simulink model "Assignment_1"  (R2022b)
settings: Solver=FixedStepAuto  StartTime=0.0  StopTime=10.0  FixedStep=1e-3  RelTol=1e-3  EnableMultiTasking=on
undefined symbols (not defined in the file): D0, D1, D10, D11, D12, D13, D2, D3, D5, D6, D8, D9, PTA0, PTA1, PTA2, PTB9, PTC16, PTC17, PTC2, PTC4, PTD0, PTD1, PTD2, PTD3
libraries: frdmk64flib x12
settings Model: ExtModeTrigDuration=5  Creator=aldenluscher  LastModifiedBy=andre
settings OptimizationCC: EnhancedBackFolding=on  PassReuseOutputArgsAs=Individual arguments  ZeroExternalMemoryAtStartup=off  ZeroInternalMemoryAtStartup=off  MaxStackSize=64  OptimizeBlockOrder=speed  DifferentSizesBufferReuse=on  OptimizationCustomize=off  EfficientTunableParamExpr=on
settings DebuggingCC: ParameterTunabilityLossMsg=error
settings HardwareCC: ProdBitPerPointer=32  ProdBitPerSizeT=32  ProdBitPerPtrDiffT=32  ProdLargestAtomicInteger=Long  ProdLargestAtomicFloat=Double  ProdWordSize=32  ProdHWDeviceType=ARM Compatible->ARM Cortex
settings SFSimCC: MATLABDynamicMemAlloc=off
settings RTWCC: Description=Embedded Coder  SystemTargetFile=ert.tlc  HardwareBoard=NXP FRDM-K64F  TLCOptions="-aInlineSetEventsForThisBaseRateFcn=TLC_FALSE -aSuppressMultiTaskScheduler=TLC_FALSE  -aRateBasedStepFcn=0"  TemplateMakefile=ert_default_tmf  Toolchain=GNU Tools for ARM Embedded Processors
settings CodeAppCC: ForceParamTrailComments=on  IgnoreCustomStorageClasses=off  OperatorAnnotations=on  SimulinkDataObjDesc=on  SFDataObjDesc=on  InsertBlockDesc=on
settings ERTTargetCC: ExtModeTransport=4  ExtModeMexFile=sendToCommService

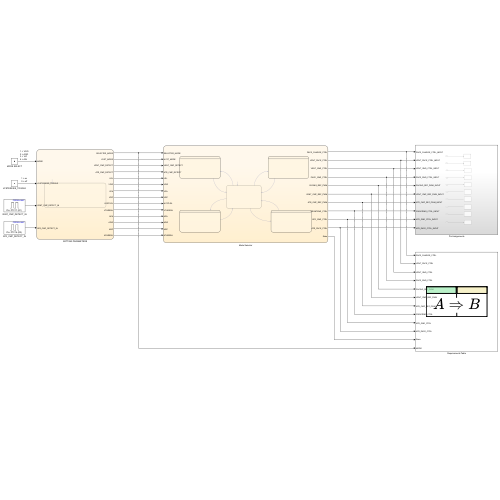
[thumbnail: Simulink's stored preview of the top-level diagram]
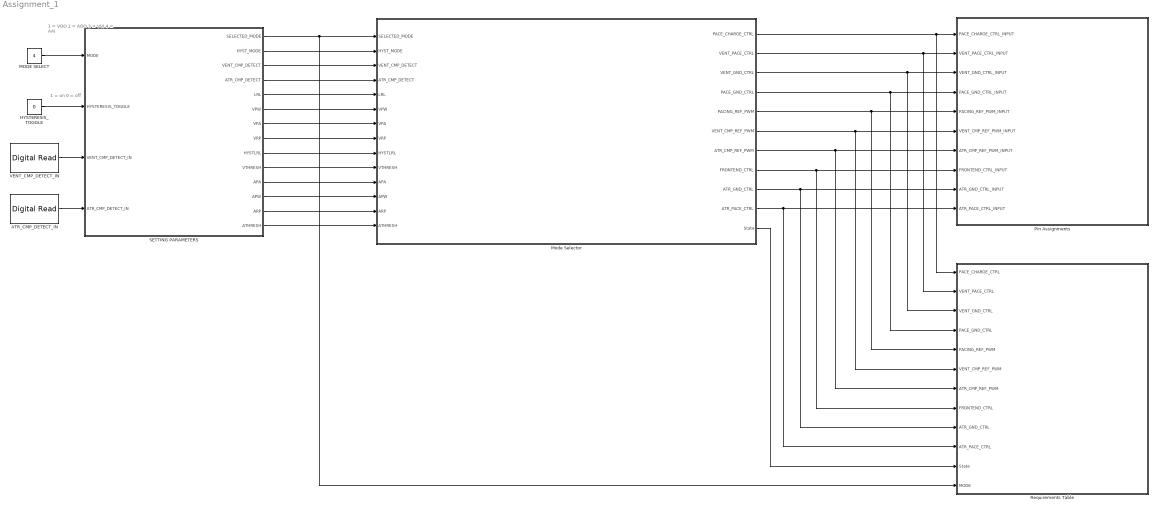
== system Assignment_1 ==
  note: 1 = VOO
      | 2 = AOO
      | 3 = VVI
      | 4 = AAI
  note: 1 = on
      | 0 = off
  ATR_CMP_DETECT_IN : frdmk64flib/Digital Read  Whichpin=PTC16 (D0)  SampleTime=-1
  HYSTERESIS_TOGGLE : Constant  Value=0
  MODE SELECT : Constant  Value=4  OutDataTypeStr=int8
  Mode Selector : Stateflow chart  TreatAsAtomicUnit=on
      settings: PortSchema="{\"entries\":[{\"content\":{\"sides\":[{\"content\":{\"connectorIds\":[\"In7\",\"In9\",\"In6\",\"In14\",\"In8\",\"In3\",\"In4\",\"In2\",\"In5\",\"In1\",\"In10\",\"In11\",\"In12\",\"In13\"]},\"type\":\"ConnectorPlacement.EquallySpacedRectSide\",\"uuid\":\"804be3be-5f9e-4b62-b5c8-dc084235daae\"},{\"content\":{\"connectorIds\":[\"Out1\",\"Out2\",\"Out3\",\"Out4\",\"Out5\",\"Out6\",\"Out11\",\"Out7\",\"Out8\",\"Out9\",\"Out10\"],\"side\":\"RIGHT\"},\"type\":\"ConnectorPlacement.EquallySpacedRectSide\",\"uuid\":\"906acfdb-1dc8-44fd-8d51-f28f98719a27\"},{\"content\":{\"connectorIds\":[],\"side\":\"TOP\"},\"type\":\"ConnectorPlacement.EquallySpacedRectSide\",\"uuid\":\"8d057b55-2cbd-487f-8484-177f9fa59c90\"}]},\"type\":\"ConnectorPlacement.EquallySpacedConnector\",\"uuid\":\"d5bd6f86-9a36-412f-a1f0-e96663509123\"}],\"packageUris\":[\"http://schema.mathworks.com/mf0/Connector/R2020b\"],\"version\":\"1.0\"}"
  Pin Assignments : Subsystem
  Requirements Table : Requirements Table  TreatAsAtomicUnit=on
  SETTING PARAMETERS : Stateflow chart  TreatAsAtomicUnit=on
      settings: PortSchema="{\"entries\":[{\"content\":{\"sides\":[{\"content\":{\"connectorIds\":[\"In1\",\"In2\",\"In3\",\"In4\"]},\"type\":\"ConnectorPlacement.EquallySpacedRectSide\",\"uuid\":\"3aca0bd7-629a-4c5c-b565-6ed0578fed9d\"},{\"content\":{\"connectorIds\":[\"Out7\",\"Out9\",\"Out6\",\"Out14\",\"Out8\",\"Out3\",\"Out4\",\"Out2\",\"Out5\",\"Out1\",\"Out10\",\"Out11\",\"Out12\",\"Out13\"],\"side\":\"RIGHT\"},\"type\":\"ConnectorPlacement.EquallySpacedRectSide\",\"uuid\":\"ab26bc13-3a59-4dfe-8b46-0847370ad477\"},{\"content\":{\"connectorIds\":[],\"side\":\"TOP\"},\"type\":\"ConnectorPlacement.EquallySpacedRectSide\",\"uuid\":\"fc5ed4b5-9a01-4cf9-a838-586958f03313\"}]},\"type\":\"ConnectorPlacement.EquallySpacedConnector\",\"uuid\":\"c620314d-9c7d-46a3-b2b8-c6bca5c5944e\"}],\"packageUris\":[\"http://schema.mathworks.com/mf0/Connector/R2020b\"],\"version\":\"1.0\"}"
  VENT_CMP_DETECT_IN : frdmk64flib/Digital Read  Whichpin=PTC17 (D1)  SampleTime=-1
  wires:
  MODE SELECT/1 -> SETTING PARAMETERS/1(MODE)
  HYSTERESIS_TOGGLE/1 -> SETTING PARAMETERS/2(HYSTERESIS_TOGGLE)
  VENT_CMP_DETECT_IN/1 -> SETTING PARAMETERS/3(VENT_CMP_DETECT_IN)
  Mode Selector/4(PACE_GND_CTRL) -> Requirements Table/4(PACE_GND_CTRL), Pin Assignments/4(PACE_GND_CTRL_INPUT)
  Mode Selector/7(FRONTEND_CTRL) -> Pin Assignments/8(FRONTEND_CTRL_INPUT), Requirements Table/8(FRONTEND_CTRL)
  Mode Selector/5(PACING_REF_PWM) -> Requirements Table/5(PACING_REF_PWM), Pin Assignments/5(PACING_REF_PWM_INPUT)
  Mode Selector/1(PACE_CHARGE_CTRL) -> Requirements Table/1(PACE_CHARGE_CTRL), Pin Assignments/1(PACE_CHARGE_CTRL_INPUT)
  Mode Selector/3(VENT_GND_CTRL) -> Requirements Table/3(VENT_GND_CTRL), Pin Assignments/3(VENT_GND_CTRL_INPUT)
  Mode Selector/6(VENT_CMP_REF_PWM) -> Requirements Table/6(VENT_CMP_REF_PWM), Pin Assignments/6(VENT_CMP_REF_PWM_INPUT)
  Mode Selector/2(VENT_PACE_CTRL) -> Requirements Table/2(VENT_PACE_CTRL), Pin Assignments/2(VENT_PACE_CTRL_INPUT)
  SETTING PARAMETERS/1(VTHRESH) -> Mode Selector/1(VTHRESH)
  SETTING PARAMETERS/2(VRP) -> Mode Selector/2(VRP)
  SETTING PARAMETERS/3(VPW) -> Mode Selector/3(VPW)
  SETTING PARAMETERS/4(VPA) -> Mode Selector/4(VPA)
  SETTING PARAMETERS/5(HYSTLRL) -> Mode Selector/5(HYSTLRL)
  SETTING PARAMETERS/6(VENT_CMP_DETECT) -> Mode Selector/6(VENT_CMP_DETECT)
  SETTING PARAMETERS/7(SELECTED_MODE) -> Requirements Table/12(MODE), Mode Selector/7(SELECTED_MODE)
  SETTING PARAMETERS/8(LRL) -> Mode Selector/8(LRL)
  SETTING PARAMETERS/9(HYST_MODE) -> Mode Selector/9(HYST_MODE)
  SETTING PARAMETERS/10(APA) -> Mode Selector/10(APA)
  SETTING PARAMETERS/11(APW) -> Mode Selector/11(APW)
  Mode Selector/8(ATR_GND_CTRL) -> Pin Assignments/9(ATR_GND_CTRL_INPUT), Requirements Table/9(ATR_GND_CTRL)
  Mode Selector/9(ATR_PACE_CTRL) -> Pin Assignments/10(ATR_PACE_CTRL_INPUT), Requirements Table/10(ATR_PACE_CTRL)
  Mode Selector/10(State) -> Requirements Table/11(State)
  ATR_CMP_DETECT_IN/1 -> SETTING PARAMETERS/4(ATR_CMP_DETECT_IN)
  SETTING PARAMETERS/12(ARP) -> Mode Selector/12(ARP)
  SETTING PARAMETERS/13(ATHRESH) -> Mode Selector/13(ATHRESH)
  SETTING PARAMETERS/14(ATR_CMP_DETECT) -> Mode Selector/14(ATR_CMP_DETECT)
  Mode Selector/11(ATR_CMP_REF_PWM) -> Requirements Table/7(ATR_CMP_REF_PWM), Pin Assignments/7(ATR_CMP_REF_PWM_INPUT)

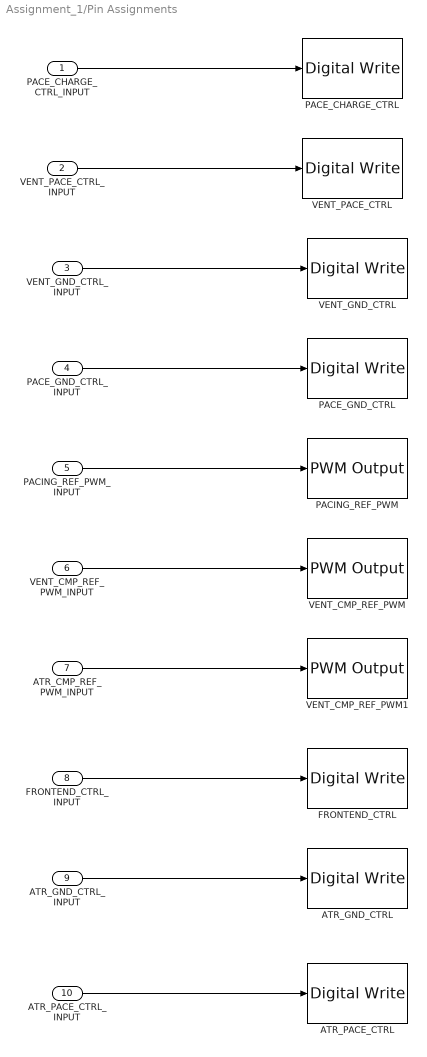
== system Assignment_1/Pin Assignments ==
  PACE_CHARGE_CTRL_INPUT : Inport
  VENT_PACE_CTRL_INPUT : Inport  Port=2
  VENT_GND_CTRL_INPUT : Inport  Port=3
  PACE_GND_CTRL_INPUT : Inport  Port=4
  PACING_REF_PWM_INPUT : Inport  Port=5
  VENT_CMP_REF_PWM_INPUT : Inport  Port=6
  ATR_CMP_REF_PWM_INPUT : Inport  Port=7
  FRONTEND_CTRL_INPUT : Inport  Port=8
  ATR_GND_CTRL_INPUT : Inport  Port=9
  ATR_PACE_CTRL_INPUT : Inport  Port=10
  ATR_GND_CTRL : frdmk64flib/Digital Write  Whichpin=PTD2 (D11)
  ATR_PACE_CTRL : frdmk64flib/Digital Write  Whichpin=PTA0 (D8)
  FRONTEND_CTRL : frdmk64flib/Digital Write  Whichpin=PTD1 (D13)
  PACE_CHARGE_CTRL : frdmk64flib/Digital Write  Whichpin=PTB9 (D2)
  PACE_GND_CTRL : frdmk64flib/Digital Write  Whichpin=PTD0 (D10)
  PACING_REF_PWM : frdmk64flib/PWM Output  Whichpin=PTA2 (D5)  InitialFrequency=2000  InitialDutyCycle=0
  VENT_CMP_REF_PWM : frdmk64flib/PWM Output  Whichpin=PTA1 (D3)  InitialFrequency=2000  InitialDutyCycle=0
  VENT_CMP_REF_PWM1 : frdmk64flib/PWM Output  Whichpin=PTC2 (D6)  InitialFrequency=2000  InitialDutyCycle=0
  VENT_GND_CTRL : frdmk64flib/Digital Write  Whichpin=PTD3 (D12)
  VENT_PACE_CTRL : frdmk64flib/Digital Write  Whichpin=PTC4 (D9)
  wires:
  VENT_PACE_CTRL_INPUT/1 -> VENT_PACE_CTRL/1
  PACE_GND_CTRL_INPUT/1 -> PACE_GND_CTRL/1
  PACE_CHARGE_CTRL_INPUT/1 -> PACE_CHARGE_CTRL/1
  PACING_REF_PWM_INPUT/1 -> PACING_REF_PWM/1
  VENT_GND_CTRL_INPUT/1 -> VENT_GND_CTRL/1
  VENT_CMP_REF_PWM_INPUT/1 -> VENT_CMP_REF_PWM/1
  FRONTEND_CTRL_INPUT/1 -> FRONTEND_CTRL/1
  ATR_GND_CTRL_INPUT/1 -> ATR_GND_CTRL/1
  ATR_PACE_CTRL_INPUT/1 -> ATR_PACE_CTRL/1
  ATR_CMP_REF_PWM_INPUT/1 -> VENT_CMP_REF_PWM1/1

== stateflow chart Assignment_1/SETTING PARAMETERS ==
  state Parameters_
    SELECTED_MODE = MODE; % Pacing Mode
    HYST_MODE = HYSTERESIS_TOGGLE; % Toggles On/Off Hysteresis (1 = on, 0 = off)
    VENT_CMP_DETECT = VENT_CMP_DETECT_IN; % Input value read from D1 pin
    ATR_CMP_DETECT = ATR_CMP_DETECT_IN;% Input value read from D0 pin
    LRL = 120; %  Lower Rate Limit (e.g. 120ppm)
    HYSTLRL = 50; % Ventricle Hysteresis Lower Rate Limit (e.g. 50ppm)
    VPW = 1; % Ventricle Pulse Width
    VPA = 3.5; % Ventricle Pulse Amplitude (as voltage from 1-5V)
    VRP = 300; % Ventricle Refractory Period (msec)
    VTHRESH = 70; % Ventricle Pulse Detection Threshold as PWM Value (e.g 70% of 5V)
    APW = 1; % Atrial Pulse Width
    APA = 3.5; % Atrial Pulse Amplitude (as voltage from 1-5V)
    ARP = 300; % Atrial Refractory Period (msec)
    ATHRESH = 70; % Atrial Pulse Detection Threshold as a PWM Value (e.g. 70% of 5V)
  (default) -> Parameters_
  data: PACING_PERIOD local; MODE input int8 [1..4]; HYSTERESIS_TOGGLE input; VENT_CMP_DETECT_IN input; VTHRESH output; VRP output; VPW output; VPA output; HYSTLRL output; VENT_CMP_DETECT output; SELECTED_MODE output; LRL output; HYST_MODE output; APA output; APW output; ATR_CMP_DETECT_IN input; ARP output; ATHRESH output; ATR_CMP_DETECT output

== stateflow chart Assignment_1/Requirements Table ==
  (default) -> (junction 1073752893)
  (junction 1073752893) -> (junction 1073752894) : {
      | % SF_REQ_REV_07
      | }
  (junction 1073752894) -> (junction 1073752896) : {
      | % HEADER_ASSIGNMENTS
      |
      | }
  (junction 1073752896) -> (junction 1073752898) : {
      | % START_A_4
      | }
  (junction 1073752898) -> (junction 1073752900) : {
      | }
  (junction 1073752900) -> (junction 1073752902) : {
      | reqtable_assumption((0<= State && State <= 2), 4);
      | }
  (junction 1073752902) -> (junction 1073752904) : {
      | }
  (junction 1073752904) -> (junction 1073752906) : {
      | % END_A_4
      | }
  (junction 1073752906) -> (junction 1073753176) : {
      | % START_A_76
      | }
  (junction 1073753176) -> (junction 1073753178) : {
      | }
  (junction 1073753178) -> (junction 1073753180) : {
      | reqtable_assumption((1<= MODE && MODE <= 4), 76);
      | }
  (junction 1073753180) -> (junction 1073753182) : {
      | }
  (junction 1073753182) -> (junction 1073753184) : {
      | % END_A_76
      | }
  (junction 1073753184) -> (junction 1073752908) : {
      | % START_R_40
      | }
  (junction 1073752908) -> (junction 1073752910) : {
      | }
  (junction 1073752910) -> (junction 1073752912)
  (junction 1073752912) -> (junction 1073752914) [order 1] : [(((MODE) == (1)))]
  (junction 1073752912) -> (junction 1073752956) [order 2]
  (junction 1073752914) -> (junction 1073752916) : {
      | reqtable_postcondition((((ATR_PACE_CTRL) == (0))) && (((ATR_GND_CTRL) == (0))) && (((PACING_REF_PWM) >= (0) && (PACING_REF_PWM) <= (100))) && (((VENT_CMP_REF_PWM) >= (0) && (VENT_CMP_REF_PWM) <= (100))) && (((ATR_CMP_REF_PWM) >= (0) && (ATR_CMP_REF_PWM) <= (100))) && (((FRONTEND_CTRL) == (0))), 'R:1');
      |
      |
      | }
  (junction 1073752916) -> (junction 1073752918) : {
      | }
  (junction 1073752918) -> (junction 1073752920) : {
      | % START_R_16
      | }
  (junction 1073752920) -> (junction 1073752922) : {
      | }
  (junction 1073752922) -> (junction 1073752924)
  (junction 1073752924) -> (junction 1073752926) [order 1] : [(((State) == (0)))]
  (junction 1073752924) -> (junction 1073752932) [order 2]
  (junction 1073752926) -> (junction 1073752928) : {
      | reqtable_postcondition((((PACE_CHARGE_CTRL) == (1))) && (((PACE_GND_CTRL) == (1))) && (((VENT_PACE_CTRL) == (0))) && (((VENT_GND_CTRL) == (1))), 'R:1.1');
      |
      |
      | }
  (junction 1073752928) -> (junction 1073752930) : {
      | }
  (junction 1073752930) -> (junction 1073752932)
  (junction 1073752932) -> (junction 1073752934)
  (junction 1073752934) -> (junction 1073752936) : {
      | % END_R_16
      | }
  (junction 1073752936) -> (junction 1073752938) : {
      | % START_R_22
      | }
  (junction 1073752938) -> (junction 1073752940) : {
      | }
  (junction 1073752940) -> (junction 1073752942)
  (junction 1073752942) -> (junction 1073752944) [order 1] : [(((State) == (1)))]
  (junction 1073752942) -> (junction 1073752950) [order 2]
  (junction 1073752944) -> (junction 1073752946) : {
      | reqtable_postcondition((((PACE_CHARGE_CTRL) == (0))) && (((PACE_GND_CTRL) == (1))) && (((VENT_PACE_CTRL) == (1))) && (((VENT_GND_CTRL) == (0))), 'R:1.2');
      |
      |
      | }
  (junction 1073752946) -> (junction 1073752948) : {
      | }
  (junction 1073752948) -> (junction 1073752950)
  (junction 1073752950) -> (junction 1073752952)
  (junction 1073752952) -> (junction 1073752954) : {
      | % END_R_22
      | }
  (junction 1073752954) -> (junction 1073752956)
  (junction 1073752956) -> (junction 1073752958)
  (junction 1073752958) -> (junction 1073752960) : {
      | % END_R_40
      | }
  (junction 1073752960) -> (junction 1073752962) : {
      | % START_R_43
      | }
  (junction 1073752962) -> (junction 1073752964) : {
      | }
  (junction 1073752964) -> (junction 1073752966)
  (junction 1073752966) -> (junction 1073752968) [order 1] : [(((MODE) == (2)))]
  (junction 1073752966) -> (junction 1073753010) [order 2]
  (junction 1073752968) -> (junction 1073752970) : {
      | reqtable_postcondition((((VENT_PACE_CTRL) == (0))) && (((VENT_GND_CTRL) == (0))) && (((PACING_REF_PWM) >= (0) && (PACING_REF_PWM) <= (100))) && (((VENT_CMP_REF_PWM) >= (0) && (VENT_CMP_REF_PWM) <= (100))) && (((ATR_CMP_REF_PWM) >= (0) && (ATR_CMP_REF_PWM) <= (100))) && (((FRONTEND_CTRL) == (0))), 'R:2');
      |
      |
      | }
  (junction 1073752970) -> (junction 1073752972) : {
      | }
  (junction 1073752972) -> (junction 1073752974) : {
      | % START_R_25
      | }
  (junction 1073752974) -> (junction 1073752976) : {
      | }
  (junction 1073752976) -> (junction 1073752978)
  (junction 1073752978) -> (junction 1073752980) [order 1] : [(((State) == (0)))]
  (junction 1073752978) -> (junction 1073752986) [order 2]
  (junction 1073752980) -> (junction 1073752982) : {
      | reqtable_postcondition((((PACE_CHARGE_CTRL) == (1))) && (((PACE_GND_CTRL) == (1))) && (((ATR_PACE_CTRL) == (0))) && (((ATR_GND_CTRL) == (1))), 'R:2.1');
      |
      |
      | }
  (junction 1073752982) -> (junction 1073752984) : {
      | }
  (junction 1073752984) -> (junction 1073752986)
  (junction 1073752986) -> (junction 1073752988)
  (junction 1073752988) -> (junction 1073752990) : {
      | % END_R_25
      | }
  (junction 1073752990) -> (junction 1073752992) : {
      | % START_R_28
      | }
  (junction 1073752992) -> (junction 1073752994) : {
      | }
  (junction 1073752994) -> (junction 1073752996)
  (junction 1073752996) -> (junction 1073752998) [order 1] : [(((State) == (1)))]
  (junction 1073752996) -> (junction 1073753004) [order 2]
  (junction 1073752998) -> (junction 1073753000) : {
      | reqtable_postcondition((((PACE_CHARGE_CTRL) == (0))) && (((PACE_GND_CTRL) == (1))) && (((ATR_PACE_CTRL) == (1))) && (((ATR_GND_CTRL) == (0))), 'R:2.2');
      |
      |
      | }
  (junction 1073753000) -> (junction 1073753002) : {
      | }
  (junction 1073753002) -> (junction 1073753004)
  (junction 1073753004) -> (junction 1073753006)
  (junction 1073753006) -> (junction 1073753008) : {
      | % END_R_28
      | }
  (junction 1073753008) -> (junction 1073753010)
  (junction 1073753010) -> (junction 1073753012)
  (junction 1073753012) -> (junction 1073753014) : {
      | % END_R_43
      | }
  (junction 1073753014) -> (junction 1073753016) : {
      | % START_R_61
      | }
  (junction 1073753016) -> (junction 1073753018) : {
      | }
  (junction 1073753018) -> (junction 1073753020)
  (junction 1073753020) -> (junction 1073753022) [order 1] : [(((MODE) == (3)))]
  (junction 1073753020) -> (junction 1073753082) [order 2]
  (junction 1073753022) -> (junction 1073753024) : {
      | reqtable_postcondition((((ATR_PACE_CTRL) == (0))) && (((ATR_GND_CTRL) == (0))) && (((PACING_REF_PWM) >= (0) && (PACING_REF_PWM) <= (100))) && (((VENT_CMP_REF_PWM) >= (0) && (VENT_CMP_REF_PWM) <= (100))) && (((ATR_CMP_REF_PWM) >= (0) && (ATR_CMP_REF_PWM) <= (100))) && (((FRONTEND_CTRL) == (1))), 'R:3');
      |
      |
      | }
  (junction 1073753024) -> (junction 1073753026) : {
      | }
  (junction 1073753026) -> (junction 1073753028) : {
      | % START_R_64
      | }
  (junction 1073753028) -> (junction 1073753030) : {
      | }
  (junction 1073753030) -> (junction 1073753032)
  (junction 1073753032) -> (junction 1073753034) [order 1] : [(((State) == (0)))]
  (junction 1073753032) -> (junction 1073753040) [order 2]
  (junction 1073753034) -> (junction 1073753036) : {
      | reqtable_postcondition((((PACE_CHARGE_CTRL) == (1))) && (((PACE_GND_CTRL) == (1))) && (((VENT_PACE_CTRL) == (0))) && (((VENT_GND_CTRL) == (1))), 'R:3.1');
      |
      |
      | }
  (junction 1073753036) -> (junction 1073753038) : {
      | }
  (junction 1073753038) -> (junction 1073753040)
  (junction 1073753040) -> (junction 1073753042)
  (junction 1073753042) -> (junction 1073753044) : {
      | % END_R_64
      | }
  (junction 1073753044) -> (junction 1073753046) : {
      | % START_R_67
      | }
  (junction 1073753046) -> (junction 1073753048) : {
      | }
  (junction 1073753048) -> (junction 1073753050)
  (junction 1073753050) -> (junction 1073753052) [order 1] : [(((State) == (1)))]
  (junction 1073753050) -> (junction 1073753058) [order 2]
  (junction 1073753052) -> (junction 1073753054) : {
      | reqtable_postcondition((((PACE_CHARGE_CTRL) == (0))) && (((PACE_GND_CTRL) == (1))) && (((VENT_PACE_CTRL) == (1))) && (((VENT_GND_CTRL) == (0))), 'R:3.2');
      |
      |
      | }
  (junction 1073753054) -> (junction 1073753056) : {
      | }
  (junction 1073753056) -> (junction 1073753058)
  (junction 1073753058) -> (junction 1073753060)
  (junction 1073753060) -> (junction 1073753062) : {
      | % END_R_67
      | }
  (junction 1073753062) -> (junction 1073753064) : {
      | % START_R_73
      | }
  (junction 1073753064) -> (junction 1073753066) : {
      | }
  (junction 1073753066) -> (junction 1073753068)
  (junction 1073753068) -> (junction 1073753070) [order 1] : [(((State) == (2)))]
  (junction 1073753068) -> (junction 1073753076) [order 2]
  (junction 1073753070) -> (junction 1073753072) : {
      | reqtable_postcondition((((PACE_CHARGE_CTRL) == (1))) && (((PACE_GND_CTRL) == (1))) && (((VENT_PACE_CTRL) == (0))) && (((VENT_GND_CTRL) == (1))), 'R:3.3');
      |
      |
      | }
  (junction 1073753072) -> (junction 1073753074) : {
      | }
  (junction 1073753074) -> (junction 1073753076)
  (junction 1073753076) -> (junction 1073753078)
  (junction 1073753078) -> (junction 1073753080) : {
      | % END_R_73
      | }
  (junction 1073753080) -> (junction 1073753082)
  (junction 1073753082) -> (junction 1073753084)
  (junction 1073753084) -> (junction 1073753086) : {
      | % END_R_61
      | }
  (junction 1073753086) -> (junction 1073753088) : {
      | % START_R_52
      | }
  (junction 1073753088) -> (junction 1073753090) : {
      | }
  (junction 1073753090) -> (junction 1073753092)
  (junction 1073753092) -> (junction 1073753094) [order 1] : [(((MODE) == (4)))]
  (junction 1073753092) -> (junction 1073753154) [order 2]
  (junction 1073753094) -> (junction 1073753096) : {
      | reqtable_postcondition((((VENT_PACE_CTRL) == (0))) && (((VENT_GND_CTRL) == (0))) && (((PACING_REF_PWM) >= (0) && (PACING_REF_PWM) <= (100))) && (((VENT_CMP_REF_PWM) >= (0) && (VENT_CMP_REF_PWM) <= (100))) && (((ATR_CMP_REF_PWM) >= (0) && (ATR_CMP_REF_PWM) <= (100))) && (((FRONTEND_CTRL) == (1))), 'R:4');
      |
      |
      | }
  (junction 1073753096) -> (junction 1073753098) : {
      | }
  (junction 1073753098) -> (junction 1073753100) : {
      | % START_R_55
      | }
  (junction 1073753100) -> (junction 1073753102) : {
      | }
  (junction 1073753102) -> (junction 1073753104)
  (junction 1073753104) -> (junction 1073753106) [order 1] : [(((State) == (0)))]
  (junction 1073753104) -> (junction 1073753112) [order 2]
  (junction 1073753106) -> (junction 1073753108) : {
      | reqtable_postcondition((((PACE_CHARGE_CTRL) == (1))) && (((PACE_GND_CTRL) == (1))) && (((ATR_PACE_CTRL) == (0))) && (((ATR_GND_CTRL) == (1))), 'R:4.1');
      |
      |
      | }
  (junction 1073753108) -> (junction 1073753110) : {
      | }
  (junction 1073753110) -> (junction 1073753112)
  (junction 1073753112) -> (junction 1073753114)
  (junction 1073753114) -> (junction 1073753116) : {
      | % END_R_55
      | }
  (junction 1073753116) -> (junction 1073753118) : {
      | % START_R_58
      | }
  (junction 1073753118) -> (junction 1073753120) : {
      | }
  (junction 1073753120) -> (junction 1073753122)
  (junction 1073753122) -> (junction 1073753124) [order 1] : [(((State) == (1)))]
  (junction 1073753122) -> (junction 1073753130) [order 2]
  (junction 1073753124) -> (junction 1073753126) : {
      | reqtable_postcondition((((PACE_CHARGE_CTRL) == (0))) && (((PACE_GND_CTRL) == (1))) && (((ATR_PACE_CTRL) == (1))) && (((ATR_GND_CTRL) == (0))), 'R:4.2');
      |
      |
      | }
  (junction 1073753126) -> (junction 1073753128) : {
      | }
  (junction 1073753128) -> (junction 1073753130)
  (junction 1073753130) -> (junction 1073753132)
  (junction 1073753132) -> (junction 1073753134) : {
      | % END_R_58
      | }
  (junction 1073753134) -> (junction 1073753136) : {
      | % START_R_70
      | }
  (junction 1073753136) -> (junction 1073753138) : {
      | }
  (junction 1073753138) -> (junction 1073753140)
  (junction 1073753140) -> (junction 1073753142) [order 1] : [(((State) == (2)))]
  (junction 1073753140) -> (junction 1073753148) [order 2]
  (junction 1073753142) -> (junction 1073753144) : {
      | reqtable_postcondition((((PACE_CHARGE_CTRL) == (1))) && (((PACE_GND_CTRL) == (1))) && (((ATR_PACE_CTRL) == (0))) && (((ATR_GND_CTRL) == (1))), 'R:4.3');
      |
      |
      | }
  (junction 1073753144) -> (junction 1073753146) : {
      | }
  (junction 1073753146) -> (junction 1073753148)
  (junction 1073753148) -> (junction 1073753150)
  (junction 1073753150) -> (junction 1073753152) : {
      | % END_R_70
      | }
  (junction 1073753152) -> (junction 1073753154)
  (junction 1073753154) -> (junction 1073753156)
  (junction 1073753156) -> (junction 1073753158) : {
      | % END_R_52
      | }
  data: PACE_CHARGE_CTRL input; VENT_PACE_CTRL input; VENT_GND_CTRL input; PACE_GND_CTRL input; PACING_REF_PWM input; VENT_CMP_REF_PWM input; ATR_CMP_REF_PWM input; FRONTEND_CTRL input; ATR_GND_CTRL input; ATR_PACE_CTRL input; State input int8 [0..2]; MODE input

== stateflow chart Assignment_1/Mode Selector ==
  state VOO
    state Pacing_
      PACE_CHARGE_CTRL = 0;
      PACE_GND_CTRL = 1;
      VENT_GND_CTRL = 0;
      VENT_PACE_CTRL = 1;
      State = 1;
    state Charging_
      State = 0;
      PACING_REF_PWM = 100*(VPA/5); % Ventricular Pulse Amplitude
      PACING_PERIOD = (60000/LRL); % Pacing Period
      PACE_CHARGE_CTRL = 1;
      PACE_GND_CTRL = 1;
      VENT_GND_CTRL = 1;
      VENT_PACE_CTRL = 0;
      ATR_PACE_CTRL = 0;
      ATR_GND_CTRL = 0;
    (default) -> VOO.Charging_
    VOO.Charging_ -> VOO.Pacing_ : after(PACING_PERIOD-VPW,msec)
        | %Charging time = Pacing Period - Pulse Width
    VOO.Pacing_ -> VOO.Charging_ : after(VPW,msec)
        | %Pacing time = Ventricle Pulse Width
  state VVI
    state Timing_Natural_PW_in_msec_
      NAT_PW=NAT_PW+1;
    state Refractory_Period_
      PACE_CHARGE_CTRL = 1;
      PACE_GND_CTRL = 1;
      VENT_GND_CTRL = 1;
      VENT_PACE_CTRL = 0;
      State = 2;
    state Charging_
      PACING_REF_PWM = 100*(VPA/5); %Pulse Amplitude
      PACING_PERIOD = (60000/LRL); %Normal Pacing Period
      HYST_PERIOD = (60000/HYSTLRL); %Hysteresis Pacing Period
      PACE_CHARGE_CTRL = 1;
      PACE_GND_CTRL = 1;
      VENT_GND_CTRL = 1;
      VENT_PACE_CTRL = 0;
      VENT_CMP_REF_PWM = VTHRESH; % Ventricle Sensing Threshold
      FRONTEND_CTRL = 1; %Sensing On
      NAT_PW = 0; % Natural Pulse Width
      TOTAL_NAT_PW = 0; % Sum of Natural Pulse
      PACE_PW = 0; % Pacemaker Pulse Width
      ARTIFICIAL = 0; % Flag to determine if a pulse was natural or artificial,
      % only has an effect when hysteresis is enabled
      State = 0;
    state Pacing_
      PACE_CHARGE_CTRL = 0;
      PACE_GND_CTRL = 1;
      VENT_GND_CTRL = 0;
      VENT_PACE_CTRL = 1;
      State = 1;
    state Setting_Initial_Period_
      PERIOD = (60000/LRL);
      % Period for each
      % pulse, initally set to the
      % normal PACING_PERIOD
      % but can be re-assigned to
      % the HYST_PERIOD if
      % hysteresis is enabled and
      % triggered
      ATR_PACE_CTRL = 0;
      ATR_GND_CTRL = 0;
      % Set ATR_PACE and
      % GND_CTRL to disabled
      % incase they were left enabled
      % from the last state
    VVI.Timing_Natural_PW_in_msec_ -> VVI.Timing_Natural_PW_in_msec_ [order 2] : after(1,msec)
        | % time the natural pulse in msec
    VVI.Timing_Natural_PW_in_msec_ -> VVI.Refractory_Period_ [order 1] : [VENT_CMP_DETECT==0]{TOTAL_NAT_PW = TOTAL_NAT_PW + NAT_PW}
        | % when the natural pulse ends add the pulsewidth of the natural pulse to the
        | % total pulsewidth of all natural pulses that have arrived while since we last
        | % paced the pacemaker
    VVI.Refractory_Period_ -> VVI.Timing_Natural_PW_in_msec_ [order 1] : [VENT_CMP_DETECT==1]{ARTIFICIAL = 0}
        | % if a natural pulse arrives while
        | % in the refractory period, the last pulse was not
        | % from the pulsemaker, and start timing the natural pulse
    VVI.Refractory_Period_ -> (junction 80) [order 2] : after(VRP-PACE_PW-TOTAL_NAT_PW,msec)
        | % after VRP-PACE_PW-TOTAL_NAT_PW then charge
    (junction 80) -> VVI.Charging_ [order 1] : [HYST_MODE == 1 && ARTIFICIAL == 0]{PERIOD = HYST_PERIOD}
        | % if hysteresis mode is on and the last pulse was a natural
        | % pulse then the pacing period for the next pulse is the HYST_PERIOD
    (junction 80) -> VVI.Charging_ [order 3] : [HYST_MODE==0]
        | % if hysteresis mode is off
    (junction 80) -> VVI.Charging_ [order 2] : [HYST_MODE == 1 && ARTIFICIAL == 1]{PERIOD = PACING_PERIOD}
        | % if hysteresis mode is on and the last pulse was sent
        | % by the pacemaker then the next pulse is the normal PACING_PERIOD
    (junction 77) -> VVI.Refractory_Period_ [order 2] : [VENT_CMP_DETECT == 1]
        | % if an incoming pulse is detected
    VVI.Pacing_ -> VVI.Refractory_Period_ : after(VPW,msec){PACE_PW = VPW, ARTIFICIAL = 1}
        | % pace for duration of VPW
    (default) -> VVI.Setting_Initial_Period_
    VVI.Charging_ -> (junction 77)
    (junction 77) -> VVI.Pacing_ [order 1] : after(PERIOD-VPW-VRP,msec)[VENT_CMP_DETECT == 0]
        | % after PERIOD-VPW-VRP if no pulse is detected then pace
    VVI.Setting_Initial_Period_ -> VVI.Charging_
  state PACING_MODE_ENTRY_POINT_
    % Selects which mode to enter into
  state AOO
    state Pacing_
      PACE_CHARGE_CTRL = 0;
      PACE_GND_CTRL = 1;
      ATR_GND_CTRL = 0;
      ATR_PACE_CTRL = 1;
      State = 1;
    state Charging_
      PACING_REF_PWM = 100*(APA/5); % Atrial Pulse Amplitude
      PACING_PERIOD = (60000/LRL); % Pacing Period
      PACE_CHARGE_CTRL = 1;
      PACE_GND_CTRL = 1;
      ATR_GND_CTRL = 1;
      ATR_PACE_CTRL = 0;
      VENT_GND_CTRL = 0;
      VENT_PACE_CTRL = 0;
      State = 0;
    (default) -> AOO.Charging_
    AOO.Charging_ -> AOO.Pacing_ : after(PACING_PERIOD-APW,msec)
        | %Charging time = Pacing Period - Pulse Width
    AOO.Pacing_ -> AOO.Charging_ : after(APW,msec)
        | %Pacing time = Atrial Pulse Width
  state AAI
    state Timing_Natural_PW_in_msec_
      NAT_PW=NAT_PW+1;
    state Refractory_Period_
      PACE_CHARGE_CTRL = 1;
      PACE_GND_CTRL = 1;
      ATR_GND_CTRL = 1;
      ATR_PACE_CTRL = 0;
      State = 2;
    state Charging_
      PACING_REF_PWM = 100*(APA/5); %Pulse Amplitude
      PACING_PERIOD = (60000/LRL); %Normal Pacing Period
      HYST_PERIOD = (60000/HYSTLRL); %Hysteresis Pacing Period
      PACE_CHARGE_CTRL = 1;
      PACE_GND_CTRL = 1;
      ATR_GND_CTRL = 1;
      ATR_PACE_CTRL = 0;
      ATR_CMP_REF_PWM = ATHRESH; % Atrial Sensing Threshold
      FRONTEND_CTRL = 1; %Sensing On
      NAT_PW = 0; % Natural Pulse Width
      TOTAL_NAT_PW = 0; % Sum of Natural Pulse
      PACE_PW = 0; % Pacemaker Pulse Width
      ARTIFICIAL = 0; % Flag to determine if a pulse was natural or artificial,
      % only has an effect when hysteresis is enabled
      State = 0;
    state Pacing_
      PACE_CHARGE_CTRL = 0;
      PACE_GND_CTRL = 1;
      ATR_GND_CTRL = 0;
      ATR_PACE_CTRL = 1;
      State = 1;
    state Setting_Initial_Period_
      PERIOD = (60000/LRL);
      % Period for each
      % pulse, initally set to the
      % normal PACING_PERIOD
      % but can be re-assigned to
      % the HYST_PERIOD if
      % hysteresis is enabled and
      % triggered
      VENT_PACE_CTRL = 0;
      VENT_GND_CTRL = 0;
      % Set VENT_PACE and
      % GND_CTRL to disabled
      % incase they were left enabled
      % from the last state
    AAI.Timing_Natural_PW_in_msec_ -> AAI.Timing_Natural_PW_in_msec_ [order 2] : after(1,msec)
        | % time the natural pulse in msec
    AAI.Timing_Natural_PW_in_msec_ -> AAI.Refractory_Period_ [order 1] : [ATR_CMP_DETECT==0]{TOTAL_NAT_PW = TOTAL_NAT_PW + NAT_PW}
        | % when the natural pulse ends add the pulsewidth of the natural pulse to the
        | % total pulsewidth of all natural pulses that have arrived while since we last
        | % paced the pacemaker
    AAI.Refractory_Period_ -> AAI.Timing_Natural_PW_in_msec_ [order 1] : [ATR_CMP_DETECT==1]{ARTIFICIAL = 0}
        | % if a natural pulse arrives while
        | % in the refractory period, the last pulse was not
        | % from the pulsemaker, and start timing the natural pulse
    AAI.Refractory_Period_ -> (junction 172) [order 2] : after(ARP-PACE_PW-TOTAL_NAT_PW,msec)
        | % after ARP-PACE_PW-TOTAL_NAT_PW then charge
    (junction 172) -> AAI.Charging_ [order 1] : [HYST_MODE == 1 && ARTIFICIAL == 0]{PERIOD = HYST_PERIOD}
        | % if hysteresis mode is on and the last pulse was a natural
        | % pulse then the pacing period for the next pulse is the HYST_PERIOD
    (junction 172) -> AAI.Charging_ [order 3] : [HYST_MODE==0]
        | % if hysteresis mode is off
    (junction 172) -> AAI.Charging_ [order 2] : [HYST_MODE == 1 && ARTIFICIAL == 1]{PERIOD = PACING_PERIOD}
        | % if hysteresis mode is on and the last pulse was sent
        | % by the pacemaker then the next pulse is the normal PACING_PERIOD
    (junction 173) -> AAI.Refractory_Period_ [order 2] : [ATR_CMP_DETECT == 1]
        | % if an incoming pulse is detected
    AAI.Pacing_ -> AAI.Refractory_Period_ : after(APW,msec){PACE_PW = APW, ARTIFICIAL = 1}
        | % pace for duration of APW
    (default) -> AAI.Setting_Initial_Period_
    AAI.Charging_ -> (junction 173)
    (junction 173) -> AAI.Pacing_ [order 1] : after(PERIOD-APW-ARP,msec)[ATR_CMP_DETECT == 0]
        | % after PERIOD-APW-ARP if no pulse is detected then pace
    AAI.Setting_Initial_Period_ -> AAI.Charging_
  PACING_MODE_ENTRY_POINT_ -> VOO [order 2] : [SELECTED_MODE==1]
  PACING_MODE_ENTRY_POINT_ -> VVI [order 1] : [SELECTED_MODE==3]
  VOO -> PACING_MODE_ENTRY_POINT_ : [SELECTED_MODE~=1]
  VVI -> PACING_MODE_ENTRY_POINT_ : [SELECTED_MODE~=3]
  (default) -> PACING_MODE_ENTRY_POINT_
  PACING_MODE_ENTRY_POINT_ -> AOO [order 3] : [SELECTED_MODE==2]
  AAI -> PACING_MODE_ENTRY_POINT_ : [SELECTED_MODE~=4]
  AOO -> PACING_MODE_ENTRY_POINT_ : [SELECTED_MODE~=2]
  PACING_MODE_ENTRY_POINT_ -> AAI [order 4] : [SELECTED_MODE==4]
  data: PACE_CHARGE_CTRL output int8; VENT_PACE_CTRL output int8; VENT_GND_CTRL output int8; PACE_GND_CTRL output int8; PACING_REF_PWM output; VENT_CMP_REF_PWM output; PACING_PERIOD local; PERIOD local; HYST_PERIOD local; FRONTEND_CTRL output int8; NAT_PW local; TOTAL_NAT_PW local; PACE_PW local; VTHRESH input; VRP input; VPW input; VPA input; HYSTLRL input; VENT_CMP_DETECT input; SELECTED_MODE input; LRL input; HYST_MODE input; ARTIFICIAL local; ATR_GND_CTRL output int8; ATR_PACE_CTRL output int8; APA input; APW input; State output int8 [0..2]; ARP input; ATHRESH input; ATR_CMP_DETECT input; ATR_CMP_REF_PWM output
